simulink model "test_motor_control_2016a"  (R2017b)
settings: Solver=ode45  StartTime=0.0  StopTime=0.25  RelTol=1e-3  EnableMultiTasking=on
settings Model: Creator=Matias  LastModifiedBy=tomej
settings DataIOCC: SaveFormat=Structure
settings OptimizationCC: LifeSpan=inf
settings DebuggingCC: SFUnexpectedBacktrackingDiag=warning  SFNoUnconditionalDefaultTransitionDiag=warning  SFExecutionAtInitializationDiag=none
settings CodeAppCC: StateflowObjectComments=on
settings GRTTargetCC: TargetLangStandard=C89/C90 (ANSI)  GeneratePreprocessorConditionals=Disable all
settings ConfigComp: CovMetricSettings=dw  CovHtmlReporting=on  CovSaveCumulativeToWorkspaceVar=on  CovSaveSingleToWorkspaceVar=on  CovExternalEMLEnable=off

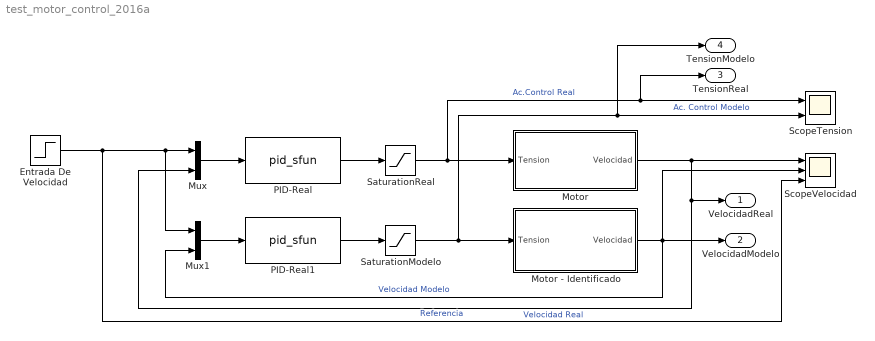
== system test_motor_control_2016a ==
  Entrada De Velocidad : Step  Time=0  After=4000  SampleTime=0
  Motor : Subsystem
  Motor - Identificado : Subsystem
  Mux : Mux  Inputs=2
  Mux1 : Mux  Inputs=2
  PID-Real : S-Function  FunctionName=pid_sfun  Parameters=0.005 25 0.00125 0.005 1/10  SFunctionDeploymentMode=off  EnableBusSupport=off
  PID-Real1 : S-Function  FunctionName=pid_sfun  Parameters=0.008 25 0.00125 0.005 1/10  SFunctionDeploymentMode=off  EnableBusSupport=off
  "SaturationModelo " : Saturate  UpperLimit=30  LowerLimit=-30
  SaturationReal : Saturate  UpperLimit=30  LowerLimit=-30
  ScopeTension : Scope  NumInputPorts=2
  ScopeVelocidad : Scope  NumInputPorts=3
  VelocidadReal : Outport
  "VelocidadModelo " : Outport  Port=2
  TensionReal : Outport  Port=3
  TensionModelo : Outport  Port=4
  wires:
  SaturationReal/1 -> Motor/1(Tension), TensionReal/1, ScopeTension/1  "Ac.Control Real"
  "SaturationModelo "/1 -> Motor - Identificado/1(Tension), TensionModelo/1, ScopeTension/2  "Ac. Control Modelo"
  Entrada De Velocidad/1 -> ScopeVelocidad/3, Mux1/1, Mux/1  "Referencia"
  PID-Real1/1 -> "SaturationModelo "/1
  Mux1/1 -> PID-Real1/1
  PID-Real/1 -> SaturationReal/1
  Mux/1 -> PID-Real/1
  Motor/1(Velocidad) -> Mux/2, VelocidadReal/1, ScopeVelocidad/1  "Velocidad Real"
  Motor - Identificado/1(Velocidad) -> "VelocidadModelo "/1, Mux1/2, ScopeVelocidad/2  "Velocidad Modelo"

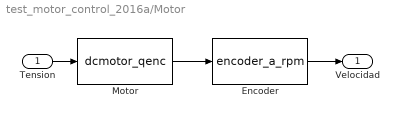
== system test_motor_control_2016a/Motor ==
  Tension : Inport
  Encoder : S-Function  FunctionName=encoder_a_rpm  Parameters=0.00001, 0.005,150  SFunctionDeploymentMode=off  EnableBusSupport=off
  Motor : S-Function  FunctionName=dcmotor_qenc  Parameters=150  SFunctionDeploymentMode=off  EnableBusSupport=off
  Velocidad : Outport
  wires:
  Motor/1 -> Encoder/1
  Encoder/1 -> Velocidad/1
  Tension/1 -> Motor/1

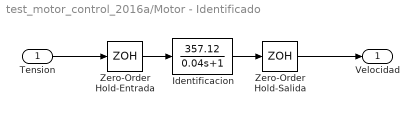
== system test_motor_control_2016a/Motor - Identificado ==
  Tension : Inport
  Identificacion : TransferFcn  Numerator=[357.12]  Denominator=[0.04 1]
  Zero-Order Hold-Entrada : ZeroOrderHold  SampleTime=0.005
  Zero-Order Hold-Salida : ZeroOrderHold  SampleTime=0.005
  Velocidad : Outport
  wires:
  Identificacion/1 -> Zero-Order Hold-Salida/1
  Zero-Order Hold-Entrada/1 -> Identificacion/1
  Zero-Order Hold-Salida/1 -> Velocidad/1
  Tension/1 -> Zero-Order Hold-Entrada/1
